simulink model "model"  (R2021b)
settings: Solver=VariableStepAuto  StartTime=0.0  StopTime=240  RelTol=1e-3
undefined symbols (not defined in the file): pK, pT
settings Model: Creator=miso  LastModifiedBy=miso

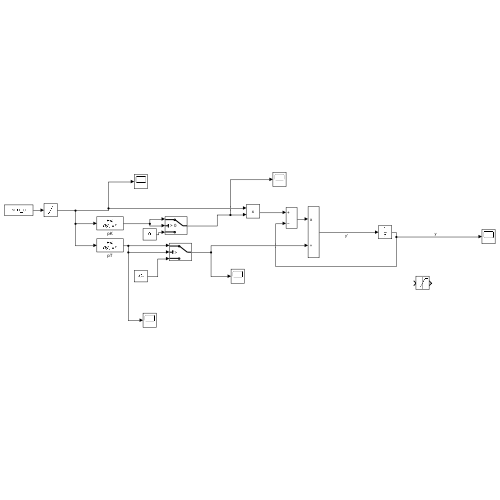
[thumbnail: Simulink's stored preview of the top-level diagram]
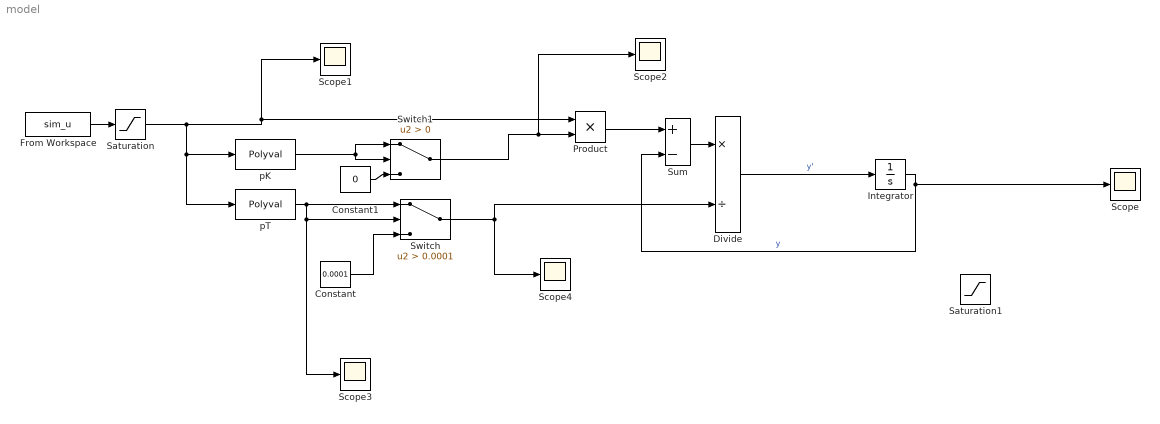
== system model ==
  Constant : Constant  Value=0.0001
  Constant1 : Constant  Value=0
  Divide : Product  Inputs=*/
  From Workspace : FromWorkspace  VariableName=sim_u
  Integrator : Integrator
  Product : Product
  Saturation : Saturate  UpperLimit=255  LowerLimit=0
  Saturation1 : Saturate  UpperLimit=1023  LowerLimit=0
  Scope{,1..4} (5 alike) : Scope
  Sum : Sum  Inputs=+-
  Switch : Switch  Criteria=u2 > Threshold  Threshold=0.0001
  Switch1 : Switch  Criteria=u2 > Threshold
  pK : Polyval  Coefs=pK
  pT : Polyval  Coefs=pT
  wires:
  Integrator/1 -> Sum/2, Scope/1  "y"
  Divide/1 -> Integrator/1  "y'"
  From Workspace/1 -> Saturation/1
  Product/1 -> Sum/1
  Sum/1 -> Divide/1
  pT/1 -> Scope3/1, Switch/2, Switch/1
  Switch/1 -> Scope4/1, Divide/2
  Constant/1 -> Switch/3
  Saturation/1 -> pT/1, pK/1, Scope1/1, Product/1
  pK/1 -> Switch1/2, Switch1/1
  Constant1/1 -> Switch1/3
  Switch1/1 -> Scope2/1, Product/2
